simulink model "untitled1"  (R2023b)
settings: Solver=VariableStepAuto  StartTime=0.0  StopTime=10.0  RelTol=1e-3
undefined symbols (not defined in the file): b, g, GR, i_0, J, Kb, Km, L, m, Q, R, Rw, tht_0, tol, v_0, wm_0, xp_0
settings Model: Creator=nikkparasar  LastModifiedBy=nikkparasar

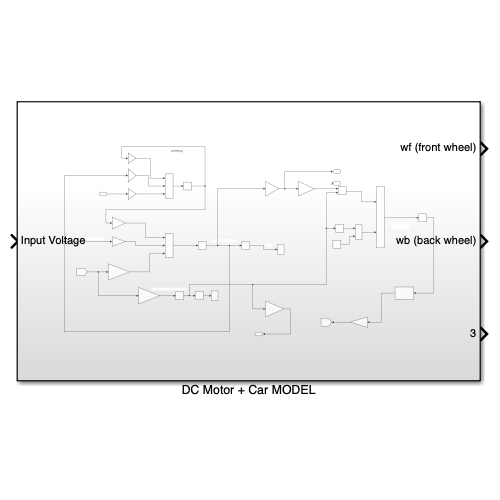
[thumbnail: Simulink's stored preview of the top-level diagram]
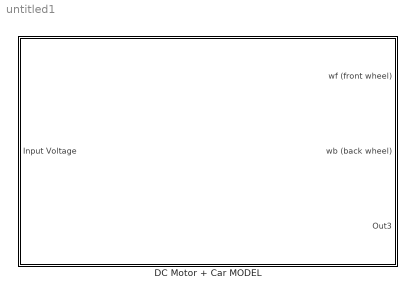
== system untitled1 ==
  DC Motor + Car MODEL : Subsystem

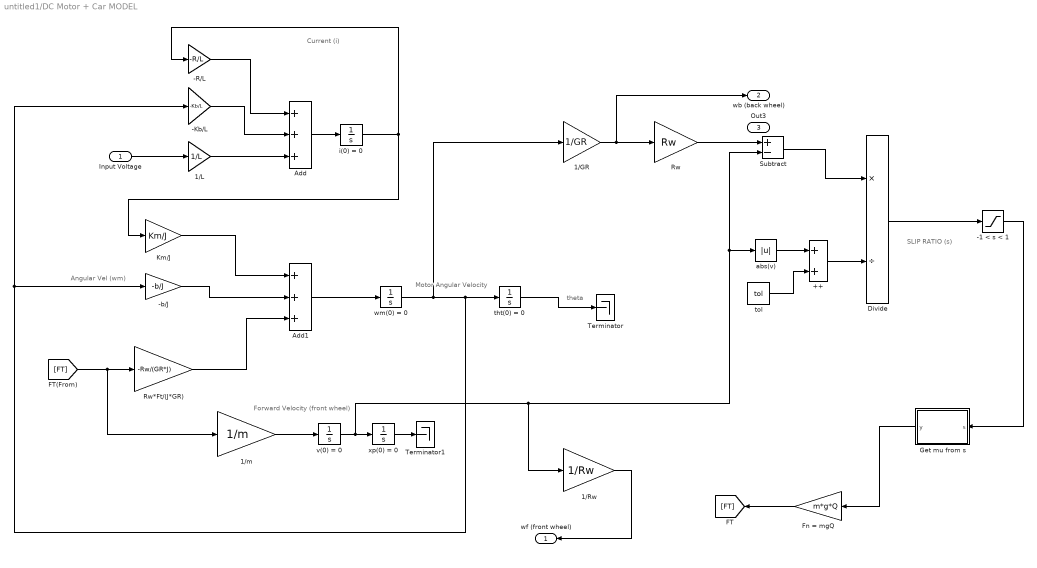
== system untitled1/DC Motor + Car MODEL ==
  note: SLIP RATIO (s)
  note: Forward Velocity (front wheel)
  note: theta
  note: Angular Vel (wm)
  note: Motor Angular Velocity
  note: Current (i)
  Input Voltage : Inport
  ++ : Sum
  -1 < s < 1 : Saturate  UpperLimit=1  LowerLimit=-1
  -Kb/L : Gain  Gain=-Kb/L
  -R/L : Gain  Gain=-R/L
  -b/J : Gain  Gain=-b/J
  1/GR : Gain  Gain=1/GR
  1/L : Gain  Gain=1/L
  1/Rw : Gain  Gain=1/Rw
  1/m : Gain  Gain=1/m
  Add : Sum  Inputs=+++
  Add1 : Sum  Inputs=+++
  Divide : Product  Inputs=*/  RndMeth=Zero  SaturateOnIntegerOverflow=on
  Fn = mgQ : Gain  Gain=m*g*Q
  Get mu from s : MATLAB Function  TreatAsAtomicUnit=on
  Km/J : Gain  Gain=Km/J
  Rw : Gain  Gain=Rw
  Rw*Ft/(J*GR) : Gain  Gain=-Rw/(GR*J)
  Subtract : Sum  Inputs=+-
  Terminator : Terminator
  Terminator1 : Terminator
  abs(v) : Abs  SaturateOnIntegerOverflow=off
  i(0) = 0 : Integrator  InitialCondition=i_0
  tht(0) = 0 : Integrator  InitialCondition=tht_0
  tol : Constant  Value=tol
  v(0) = 0 : Integrator  InitialCondition=v_0
  wm(0) = 0 : Integrator  InitialCondition=wm_0
  "xp(0) = 0 " : Integrator  InitialCondition=xp_0
  wf (front wheel) : Outport
  wb (back wheel) : Outport  Port=2
  Out3 : Outport  Port=3
  wires:
  1/Rw/1 -> wf (front wheel)/1
  Divide/1 -> -1 < s < 1/1
  Fn = mgQ/1 -> [FT]
  Add1/1 -> wm(0) = 0/1
  1/L/1 -> Add/3
  Rw*Ft/(J*GR)/1 -> Add1/3
  -Kb/L/1 -> Add/2
  tht(0) = 0/1 -> Terminator/1
  Add/1 -> i(0) = 0/1
  Input Voltage/1 -> 1/L/1
  -R/L/1 -> Add/1
  abs(v)/1 -> ++/1
  Get mu from s/1(y) -> Fn = mgQ/1
  1/m/1 -> v(0) = 0/1
  [FT] -> 1/m/1, Rw*Ft/(J*GR)/1
  ++/1 -> Divide/2
  Rw/1 -> Subtract/1
  i(0) = 0/1 -> -R/L/1, Km/J/1
  -1 < s < 1/1 -> Get mu from s/1(s)
  1/GR/1 -> wb (back wheel)/1, Rw/1
  -b/J/1 -> Add1/2
  Km/J/1 -> Add1/1
  wm(0) = 0/1 -> tht(0) = 0/1, -Kb/L/1, -b/J/1, 1/GR/1
  tol/1 -> ++/2
  v(0) = 0/1 -> 1/Rw/1, Subtract/2, abs(v)/1, "xp(0) = 0 "/1
  "xp(0) = 0 "/1 -> Terminator1/1
  Subtract/1 -> Divide/1

== matlab function untitled1/DC Motor + Car MODEL/Get mu from s ==
  data: s input; y output
function y = fcn(s)

% slip is already saturated
% ONLY DEFINED FROM 1 to -1

a1 = 1.63;
a2 = -0.9;
a3 = -0.1;

c1 = -27;
c2 = -15;

if s<0
    s = abs(s)
    mu = -(a1*(1-exp(c1*s))+a2*(1-exp(c2*s))+a3*s);
else
    mu = a1*(1-exp(c1*s))+a2*(1-exp(c2*s))+a3*s;
end

y = mu
